simulink model "chap7_14sim"  (Simulink 7.7)
settings: Solver=ode45  StartTime=0.0  StopTime=10  RelTol=1e-3
undefined symbols (not defined in the file or in its folder): denGa, denGl, numGa, numGl
libraries: simulink x1
settings Model: Creator=ljk  LastModifiedBy=ljk  ExtModeTrigMode=oneshot  ExtModeArmWhenConnect=off  ExtModeAutoUpdateStatusClock=off
settings DataIOCC: Decimation=100  LimitDataPoints=off  SaveOutput=off  SaveTime=off
settings OptimizationCC: BlockReduction=off  BooleanDataType=off  InitFltsAndDblsToZero=on
settings DebuggingCC: SaveWithParameterizedLinksMsg=none  SignalResolutionControl=TryResolveAllWithWarning  SolverPrmCheckMsg=none  MultiTaskDSMMsg=warning  MultiTaskCondExecSysMsg=none  StrictBusMsg=None
settings HardwareCC: TargetUnknown=on
settings RTWCC: IncludeERTFirstTime=on
settings GRTTargetCC: TargetFcnLib=ansi_tfl_tmw.mat

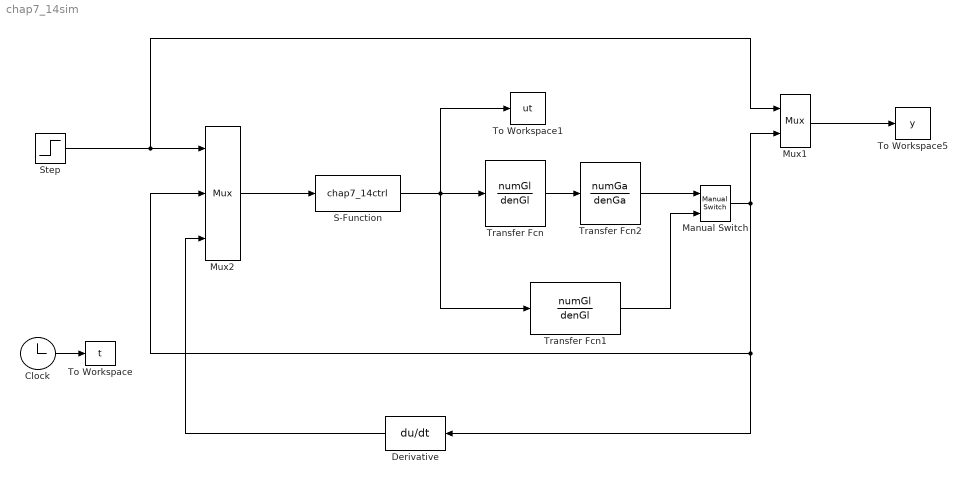
== system chap7_14sim ==
  Clock : Clock
      settings: Decimation=5
  Derivative : Derivative
  Manual Switch : simulink/Signal Routing/Manual Switch  SystemSampleTime=-1  sw=1  action=0  varsize=off
  Mux1 : Mux  Inputs=2
  Mux2 : Mux  Inputs=3
  S-Function : S-Function  FunctionName=chap7_14ctrl  EnableBusSupport=off
  Step : Step  Time=0  SampleTime=0
  To Workspace : ToWorkspace  VariableName=t  SampleTime=-1  SaveFormat=Array
  To Workspace1 : ToWorkspace  VariableName=ut  SampleTime=-1  SaveFormat=Array
  To Workspace5 : ToWorkspace  VariableName=y  SampleTime=-1  SaveFormat=Array
  Transfer Fcn : TransferFcn  Numerator=numGl  Denominator=denGl
  Transfer Fcn1 : TransferFcn  Numerator=numGl  Denominator=denGl
  Transfer Fcn2 : TransferFcn  Numerator=numGa  Denominator=denGa
  wires:
  Clock/1 -> To Workspace/1
  Step/1 -> Mux2/1, Mux1/1
  Mux2/1 -> S-Function/1
  Mux1/1 -> To Workspace5/1
  S-Function/1 -> Transfer Fcn/1, Transfer Fcn1/1, To Workspace1/1
  Derivative/1 -> Mux2/3
  Transfer Fcn1/1 -> Manual Switch/2
  Manual Switch/1 -> Mux1/2, Derivative/1, Mux2/2
  Transfer Fcn/1 -> Transfer Fcn2/1
  Transfer Fcn2/1 -> Manual Switch/1
